simulink model "GRPsimThrustUpdate"  (R2024b)
settings: Solver=VariableStepAuto  StartTime=0.0  StopTime=10.0  RelTol=1e-3
undefined symbols (not defined in the file or in its folder): factstruct
libraries: slpidlib x2, aerolibanim x1, shared6dof x1, aerolibadyn x1
settings Model: Creator=ryanmarquardt  LastModifiedBy=ryanmarquardt

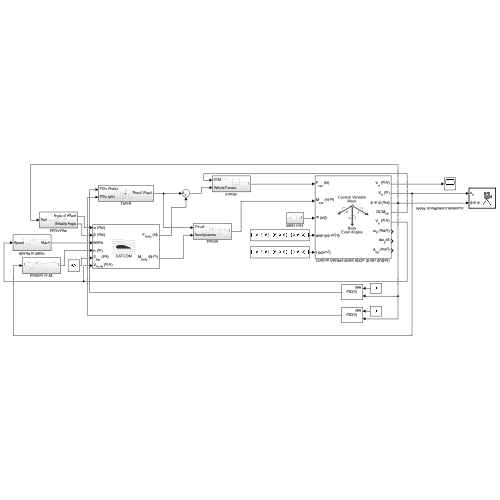
[thumbnail: Simulink's stored preview of the top-level diagram]
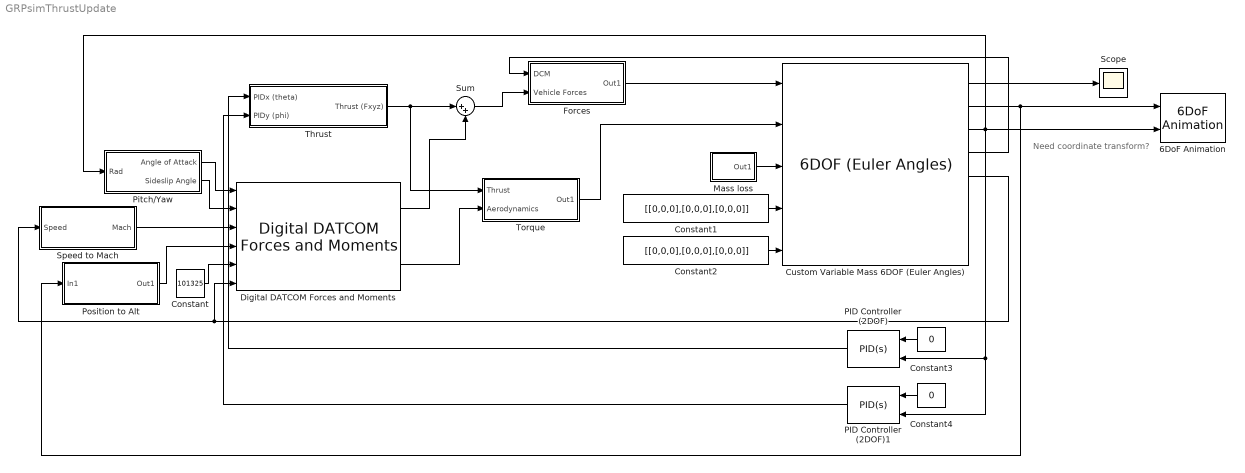
== system GRPsimThrustUpdate ==
  note: Need coordinate transform?
  6DoF Animation : aerolibanim/6DoF Animation  u1=[0 4000 -2000 2000 -5000 -3000]  u2=0.1  u3=1.0  u4=[4000 0 -5000]  u5=Fixed position  u6=[2000 500 -3150]  u7=10  u8=on
  Constant : Constant  Value=101325
  Constant1 : Constant  Value=[[0,0,0],[0,0,0],[0,0,0]]
  Constant2 : Constant  Value=[[0,0,0],[0,0,0],[0,0,0]]
  Constant3 : Constant  Value=0
  Constant4 : Constant  Value=0
  Custom Variable Mass 6DOF (Euler Angles) : shared6dof/6DOF (Euler Angles)  units=Metric (MKS)  mtype=Custom Variable  rep=Euler Angles  xme_0=[0 0 0]  Vm_0=[0 0 0]  eul_0=[0 0 0]  pm_0=[0 0 0]  mass_0=1.0  mass_e=0.5  mass_f=2.0  inertia=eye(3)  inertia_e=eye(3)  inertia_f=2*eye(3)  k_quat=1.0  vre_flag=off  abi_flag=off  aMode=0  xme_statename=''  Vm_statename=''  eul_statename=''  quat_statename=''  pm_statename=''  mass_statename=''
      settings: LibrarySourceBlock=aerolib6dof2/Custom Variable Mass 6DOF (Euler Angles)
  Digital DATCOM Forces and Moments : aerolibadyn/Digital DATCOM Forces and Moments  units=Metric (MKS)  dcase=factstruct{1}  fmode=Body  buildno=0  imethod=None - flat  emethod=None - clip  rmethod=Clip to Range  action=None
  Forces : Subsystem
  Mass loss : Subsystem
  PID Controller (2DOF) : slpidlib/PID Controller (2DOF)  Controller=PID  Form=Parallel  TimeDomain=Continuous-time  UseExternalTs=off  SampleTime=-1  IntegratorMethod=Forward Euler  FilterMethod=Forward Euler  ControllerParametersSource=internal  P=1  I=1  UseKiTs=off  D=0  UseExternalDerivativeSource=off  N=100  UseFilter=on  b=1  c=1  TunerSelectOption=Transfer Function Based (PID Tuner App)  InitialConditionSource=internal  InitialConditionForIntegrator=0  InitialConditionForFilter=0  DifferentiatorICPrevScaledInput=0  ExternalReset=none  TrackingMode=off  Kt=1  LimitOutput=off  SatLimitsSource=internal  UpperSaturationLimit=inf  LowerSaturationLimit=-inf  LinearizeAsGain=on  AntiWindupMode=none  Kb=1  LimitIntegrator=off  UpperIntegratorSaturationLimit=inf  LowerIntegratorSaturationLimit=-inf  POutMin=[]  POutMax=[]  IOutMin=[]  IOutMax=[]  DOutMin=[]  DOutMax=[]  NOutMin=[]  NOutMax=[]  bOutMin=[]  bOutMax=[]  cOutMin=[]  cOutMax=[]  SumOutMin=[]  SumOutMax=[]  SaturationOutMin=[]  SaturationOutMax=[]  PParamMin=[]  PParamMax=[]  IParamMin=[]  IParamMax=[]  DParamMin=[]  DParamMax=[]  NParamMin=[]  NParamMax=[]  bParamMin=[]  bParamMax=[]  cParamMin=[]  cParamMax=[]  KbParamMin=[]  KbParamMax=[]  KtParamMin=[]  KtParamMax=[]  KbOutMin=[]  KbOutMax=[]  KtOutMin=[]  KtOutMax=[]  IntegratorOutMin=[]  IntegratorOutMax=[]  FilterOutMin=[]  FilterOutMax=[]  SumI1OutMin=[]  SumI1OutMax=[]  SumI2OutMin=[]  SumI2OutMax=[]  SumI3OutMin=[]  SumI3OutMax=[]  SumI4OutMin=[]  SumI4OutMax=[]  SumDOutMin=[]  SumDOutMax=[]  Sum1OutMin=[]  Sum1OutMax=[]  Sum2OutMin=[]  Sum2OutMax=[]  Sum3OutMin=[]  Sum3OutMax=[]  DifferentiatorOutMin=[]  DifferentiatorOutMax=[]  FilterDiffOutCoefMin=[]  FilterDiffOutCoefMax=[]  ReciprocalOutMin=[]  ReciprocalOutMax=[]  SumDenOutMin=[]  SumDenOutMax=[]  SumNumOutMin=[]  SumNumOutMax=[]  DivideOutMin=[]  DivideOutMax=[]  UdiffTsProdOutMin=[]  UdiffTsProdOutMax=[]  NTsProdOutMin=[]  NTsProdOutMax=[]  UintegralTsProdOutMin=[]  UintegralTsProdOutMax=[]  UngainTsProdOutMin=[]  UngainTsProdOutMax=[]  ClampingZeroOutDataTypeStr=Inherit: Inherit via back propagation  ClampingZeroOutMin=[]  ClampingZeroOutMax=[]  FilterDenConstantOutDataTypeStr=Inherit: Inherit via back propagation  FilterDenConstantOutMin=[]  FilterDenConstantOutMax=[]  PCopyOutDataTypeStr=Inherit: Inherit via back propagation  PCopyOutMin=[]  PCopyOutMax=[]  NCopyOutDataTypeStr=Inherit: Inherit via back propagation  NCopyOutMin=[]  NCopyOutMax=[]  IntegratorContinuousStateAttributes=''  IntegratorStateMustResolveToSignalObject=off  IntegratorRTWStateStorageClass=Auto  FilterContinuousStateAttributes=''  FilterStateMustResolveToSignalObject=off  FilterRTWStateStorageClass=Auto  ParallelPVariant=InternalParameters  IdealPVariant=Disabled  IVariant=InternalParameters  DVariant=InternalParameters  bVariant=InternalParameters  cVariant=InternalParameters  IntegratorVariant=Continuous  SatVariant=Disabled  AWVariant=Passthrough  PCopyVariant=Disabled  TRVariant=Disabled  FdbkBlocksVariant=Forward  IdealPFdbkVariant=Disabled  SatFdbkVariant=Disabled  DerivativeFilterVariant=ContFilter  NVariant=InternalParameters  NCopyVariant=Disabled  FilterICVariant=InternalICsFilter  IntegratorICVariant=InternalICs  ExternalResetVariant=Disabled  TRSumVariant=Passthrough  SumFdbkVariant=Disabled  SumVariant=Sum_PID  TsampFilterVariant=InternalTs  TsampNgainVariant=Passthrough  TsampIntegralVariant=Disabled_SignalSpec  ExternalSaturationOutDataTypeStr=Inherit: Same as second input  DerivativeSourceVariant=ErrorSignal  PreIntVariant=InternalPreInt
  PID Controller (2DOF)1 : slpidlib/PID Controller (2DOF)  Controller=PID  Form=Parallel  TimeDomain=Continuous-time  UseExternalTs=off  SampleTime=-1  IntegratorMethod=Forward Euler  FilterMethod=Forward Euler  ControllerParametersSource=internal  P=1  I=1  UseKiTs=off  D=0  UseExternalDerivativeSource=off  N=100  UseFilter=on  b=1  c=1  TunerSelectOption=Transfer Function Based (PID Tuner App)  InitialConditionSource=internal  InitialConditionForIntegrator=0  InitialConditionForFilter=0  DifferentiatorICPrevScaledInput=0  ExternalReset=none  TrackingMode=off  Kt=1  LimitOutput=off  SatLimitsSource=internal  UpperSaturationLimit=inf  LowerSaturationLimit=-inf  LinearizeAsGain=on  AntiWindupMode=none  Kb=1  LimitIntegrator=off  UpperIntegratorSaturationLimit=inf  LowerIntegratorSaturationLimit=-inf  POutMin=[]  POutMax=[]  IOutMin=[]  IOutMax=[]  DOutMin=[]  DOutMax=[]  NOutMin=[]  NOutMax=[]  bOutMin=[]  bOutMax=[]  cOutMin=[]  cOutMax=[]  SumOutMin=[]  SumOutMax=[]  SaturationOutMin=[]  SaturationOutMax=[]  PParamMin=[]  PParamMax=[]  IParamMin=[]  IParamMax=[]  DParamMin=[]  DParamMax=[]  NParamMin=[]  NParamMax=[]  bParamMin=[]  bParamMax=[]  cParamMin=[]  cParamMax=[]  KbParamMin=[]  KbParamMax=[]  KtParamMin=[]  KtParamMax=[]  KbOutMin=[]  KbOutMax=[]  KtOutMin=[]  KtOutMax=[]  IntegratorOutMin=[]  IntegratorOutMax=[]  FilterOutMin=[]  FilterOutMax=[]  SumI1OutMin=[]  SumI1OutMax=[]  SumI2OutMin=[]  SumI2OutMax=[]  SumI3OutMin=[]  SumI3OutMax=[]  SumI4OutMin=[]  SumI4OutMax=[]  SumDOutMin=[]  SumDOutMax=[]  Sum1OutMin=[]  Sum1OutMax=[]  Sum2OutMin=[]  Sum2OutMax=[]  Sum3OutMin=[]  Sum3OutMax=[]  DifferentiatorOutMin=[]  DifferentiatorOutMax=[]  FilterDiffOutCoefMin=[]  FilterDiffOutCoefMax=[]  ReciprocalOutMin=[]  ReciprocalOutMax=[]  SumDenOutMin=[]  SumDenOutMax=[]  SumNumOutMin=[]  SumNumOutMax=[]  DivideOutMin=[]  DivideOutMax=[]  UdiffTsProdOutMin=[]  UdiffTsProdOutMax=[]  NTsProdOutMin=[]  NTsProdOutMax=[]  UintegralTsProdOutMin=[]  UintegralTsProdOutMax=[]  UngainTsProdOutMin=[]  UngainTsProdOutMax=[]  ClampingZeroOutDataTypeStr=Inherit: Inherit via back propagation  ClampingZeroOutMin=[]  ClampingZeroOutMax=[]  FilterDenConstantOutDataTypeStr=Inherit: Inherit via back propagation  FilterDenConstantOutMin=[]  FilterDenConstantOutMax=[]  PCopyOutDataTypeStr=Inherit: Inherit via back propagation  PCopyOutMin=[]  PCopyOutMax=[]  NCopyOutDataTypeStr=Inherit: Inherit via back propagation  NCopyOutMin=[]  NCopyOutMax=[]  IntegratorContinuousStateAttributes=''  IntegratorStateMustResolveToSignalObject=off  IntegratorRTWStateStorageClass=Auto  FilterContinuousStateAttributes=''  FilterStateMustResolveToSignalObject=off  FilterRTWStateStorageClass=Auto  ParallelPVariant=InternalParameters  IdealPVariant=Disabled  IVariant=InternalParameters  DVariant=InternalParameters  bVariant=InternalParameters  cVariant=InternalParameters  IntegratorVariant=Continuous  SatVariant=Disabled  AWVariant=Passthrough  PCopyVariant=Disabled  TRVariant=Disabled  FdbkBlocksVariant=Forward  IdealPFdbkVariant=Disabled  SatFdbkVariant=Disabled  DerivativeFilterVariant=ContFilter  NVariant=InternalParameters  NCopyVariant=Disabled  FilterICVariant=InternalICsFilter  IntegratorICVariant=InternalICs  ExternalResetVariant=Disabled  TRSumVariant=Passthrough  SumFdbkVariant=Disabled  SumVariant=Sum_PID  TsampFilterVariant=InternalTs  TsampNgainVariant=Passthrough  TsampIntegralVariant=Disabled_SignalSpec  ExternalSaturationOutDataTypeStr=Inherit: Same as second input  DerivativeSourceVariant=ErrorSignal  PreIntVariant=InternalPreInt
  Pitch/Yaw : Subsystem
  Position to Alt : Subsystem
  Scope : Scope
  Speed to Mach : Subsystem
  Sum : Sum  Inputs=|++
  Thrust : Subsystem
  Torque : Subsystem
  wires:
  Forces/1(Out1) -> Custom Variable Mass 6DOF (Euler Angles)/1
  Custom Variable Mass 6DOF (Euler Angles)/4 -> Forces/1(DCM)
  Sum/1 -> Forces/2(Vehicle Forces)
  Thrust/1(Thrust (Fxyz)) -> Torque/1(Thrust), Sum/1
  Digital DATCOM Forces and Moments/1 -> Sum/2
  Custom Variable Mass 6DOF (Euler Angles)/5 -> Digital DATCOM Forces and Moments/6, Speed to Mach/1(Speed)
  Constant/1 -> Digital DATCOM Forces and Moments/5
  Position to Alt/1(Out1) -> Digital DATCOM Forces and Moments/4
  PID Controller (2DOF)/1 -> Thrust/1(PIDx (theta))
  Constant2/1 -> Custom Variable Mass 6DOF (Euler Angles)/5
  Constant1/1 -> Custom Variable Mass 6DOF (Euler Angles)/4
  Custom Variable Mass 6DOF (Euler Angles)/2 -> 6DoF Animation/1, Position to Alt/1(In1)
  Pitch/Yaw/1(Angle of Attack) -> Digital DATCOM Forces and Moments/1
  Pitch/Yaw/2(Sideslip Angle) -> Digital DATCOM Forces and Moments/2
  Custom Variable Mass 6DOF (Euler Angles)/3 -> Pitch/Yaw/1(Rad), 6DoF Animation/2, PID Controller (2DOF)1/2, PID Controller (2DOF)/2
  Digital DATCOM Forces and Moments/2 -> Torque/2(Aerodynamics)
  Torque/1(Out1) -> Custom Variable Mass 6DOF (Euler Angles)/2
  Custom Variable Mass 6DOF (Euler Angles)/1 -> Scope/1
  Mass loss/1(Out1) -> Custom Variable Mass 6DOF (Euler Angles)/3
  Speed to Mach/1(Mach) -> Digital DATCOM Forces and Moments/3
  Constant4/1 -> PID Controller (2DOF)1/1
  Constant3/1 -> PID Controller (2DOF)/1
  PID Controller (2DOF)1/1 -> Thrust/2(PIDy (phi))

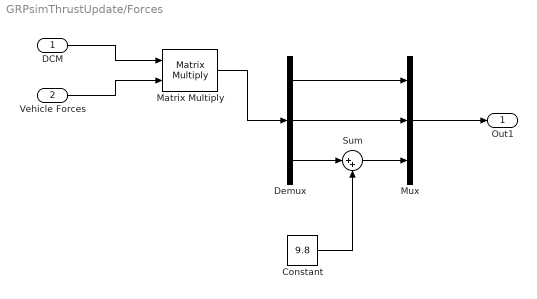
== system GRPsimThrustUpdate/Forces ==
  DCM : Inport
  Vehicle Forces : Inport  Port=2
  Constant : Constant  Value=9.8
  Demux : Demux  Outputs=3
  Matrix Multiply : Product  Multiplication=Matrix(*)
  Mux : Mux  Inputs=3
  Sum : Sum  Inputs=|++
  Out1 : Outport
  wires:
  Matrix Multiply/1 -> Demux/1
  Mux/1 -> Out1/1
  Constant/1 -> Sum/2
  Demux/3 -> Sum/1
  Demux/2 -> Mux/2
  Demux/1 -> Mux/1
  Sum/1 -> Mux/3
  DCM/1 -> Matrix Multiply/1
  Vehicle Forces/1 -> Matrix Multiply/2

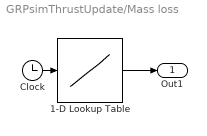
== system GRPsimThrustUpdate/Mass loss ==
  1-D Lookup Table : Lookup_n-D  NumberOfTableDimensions=1  BreakpointsForDimension1=[0;3;1000]  Table=[0.0941;0.0341;0.03]  InternalRulePriority=Speed  RndMeth=Simplest
  Clock : Clock
  Out1 : Outport
  wires:
  Clock/1 -> 1-D Lookup Table/1
  1-D Lookup Table/1 -> Out1/1

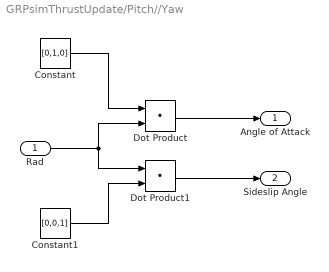
== system GRPsimThrustUpdate/Pitch//Yaw ==
  Rad : Inport
  Constant : Constant  Value=[0,1,0]
  Constant1 : Constant  Value=[0,0,1]
  Dot Product : DotProduct  OutDataTypeStr=Inherit: Inherit via internal rule
  Dot Product1 : DotProduct  OutDataTypeStr=Inherit: Inherit via internal rule
  Angle of Attack : Outport
  Sideslip Angle : Outport  Port=2
  wires:
  Constant1/1 -> Dot Product1/2
  Constant/1 -> Dot Product/1
  Rad/1 -> Dot Product/2, Dot Product1/1
  Dot Product/1 -> Angle of Attack/1
  Dot Product1/1 -> Sideslip Angle/1

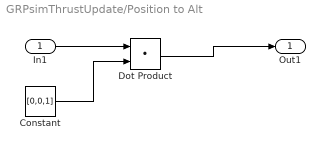
== system GRPsimThrustUpdate/Position to Alt ==
  In1 : Inport
  Constant : Constant  Value=[0,0,1]
  Dot Product : DotProduct  OutDataTypeStr=Inherit: Inherit via internal rule
  Out1 : Outport
  wires:
  In1/1 -> Dot Product/1
  Constant/1 -> Dot Product/2
  Dot Product/1 -> Out1/1

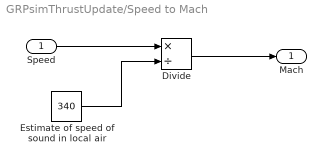
== system GRPsimThrustUpdate/Speed to Mach ==
  Speed : Inport
  Divide : Product  Inputs=*/
  Estimate of speed of sound in local air : Constant  Value=340
  Mach : Outport
  wires:
  Speed/1 -> Divide/1
  Estimate of speed of sound in local air/1 -> Divide/2
  Divide/1 -> Mach/1

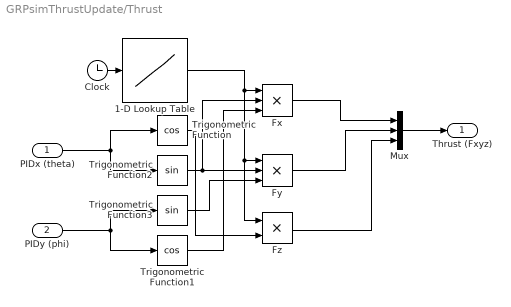
== system GRPsimThrustUpdate/Thrust ==
  PIDx (theta) : Inport
  PIDy (phi) : Inport  Port=2
  1-D Lookup Table : Lookup_n-D  NumberOfTableDimensions=1  BreakpointsForDimension1=[0;0.25;0.29999999999999999;0.5;0.75;1;1.25;1.5;1.75;2;2.25;2.5;2.75;2.8999999999999999;3]  Table=[0;30;30;20;18;17;16.5;16.5;16.25;16;16;15.75;15.5;15.5;0]  InternalRulePriority=Speed  RndMeth=Simplest
  Clock : Clock
  Fx : Product  Inputs=3
  Fy : Product  Inputs=3
  Fz : Product
  Mux : Mux  Inputs=3
  Trigonometric Function : Trigonometry  Operator=cos
  Trigonometric Function1 : Trigonometry  Operator=cos
  Trigonometric Function2 : Trigonometry
  Trigonometric Function3 : Trigonometry
  Thrust (Fxyz) : Outport
  wires:
  PIDx (theta)/1 -> Trigonometric Function2/1, Trigonometric Function/1
  1-D Lookup Table/1 -> Fz/1, Fy/1, Fx/1
  Fx/1 -> Mux/1
  Fy/1 -> Mux/2
  Mux/1 -> Thrust (Fxyz)/1
  Clock/1 -> 1-D Lookup Table/1
  PIDy (phi)/1 -> Trigonometric Function1/1, Trigonometric Function3/1
  Trigonometric Function2/1 -> Fx/2, Fy/2
  Trigonometric Function1/1 -> Fx/3
  Trigonometric Function/1 -> Fz/2
  Trigonometric Function3/1 -> Fy/3
  Fz/1 -> Mux/3

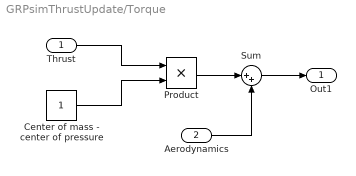
== system GRPsimThrustUpdate/Torque ==
  Thrust : Inport
  Aerodynamics : Inport  Port=2
  Center of mass - center of pressure : Constant
  Product : Product
  Sum : Sum  Inputs=|++
  Out1 : Outport
  wires:
  Sum/1 -> Out1/1
  Product/1 -> Sum/1
  Aerodynamics/1 -> Sum/2
  Center of mass - center of pressure/1 -> Product/2
  Thrust/1 -> Product/1
